simulink model "elec_a2d_sd_anti_alias_graph"  (R2020b)
settings: Solver=VariableStepAuto  StartTime=0.0  StopTime=60  MaxStep=3e-5  RelTol=1e-3  EnableMultiTasking=on
PreLoadFcn:
  | %% Global model parameters
  | fs = 1000; % A-to-D sampling rate
  | 
  | %% Filter design
  | f1 = 500; % Filter cut-off frequency
  | n = 4;    % Filter order
  | w1 = 2*pi*f1;
  | 
  | % [tmpB,tmpA] = besself(n,1); % Signal Processing Toolbox(TM)
  | tmpB = [0 0 0 0 1];
  | tmpA = [1.0000    3.1239    4.3916    3.2011    1.0000];
  | tmp_roots = roots(tmpA);
  | tcc1 = poly(tmp_roots(3:4));
  | a1 = tcc1(2);
  | b1 = tcc1(3);
  | tcc2 = poly(tmp_roots(1:2));
  | a2 = tcc2(2);
  | b2 = tcc2(3);
  | 
  | %% Filter implementation
  | R = 1e4;  % Resistance value
  | % Stage 1
  | C1 = a1/(2*b1);
  | C2 = 1/(b1*C1);
  | C1_1 = C1/( R*w1 );
  | C2_1 = C2/( R*w1 );
  | % Stage 2
  | C1 = a2/(2*b2);
  | C2 = 1/(b2*C1);
  | C1_2 = C1/( R*w1 );
  | C2_2 = C2/( R*w1 );
libraries: fl_lib x15, nesl_utility x4, ee_lib x1
CloseFcn:
  | try,close(h1_elec_a2d_sd_anti_alias),end
  | clear h1_elec_a2d_sd_anti_alias
  | 
  | 
  | clear simlog_elec_a2d_sd_anti_alias
  | clear logsout_elec_a2d_sd_anti_alias
  | clear C1 C1_1 C1_2 C2 C2_1 C2_2 R a1 a2 b1 b2 f1 fs n tcc1 tcc2 tmpA tmpB tmp_roots vOut w1
Description:
  | Analog Anti-Aliasing Filter
  | 
  | Copyright 2008-2018 The MathWorks, Inc.
settings Model: Creator=MathWorks  LastModifiedBy=dhrumilnaik
settings DataIOCC: MaxDataPoints=75000  SaveFormat=Array  SignalLoggingSaveFormat=ModelDataLogs  SaveOutput=off  SignalLogging=off  DSMLogging=off  SaveTime=off  ReturnWorkspaceOutputs=off  SignalLoggingName=logsout_elec_a2d_sd_anti_alias
settings OptimizationCC: ExpressionDepthLimit=2147483647  LifeSpan=inf
settings DebuggingCC: UnderspecifiedInitializationDetection=Classic  MergeDetectMultiDrivingBlocksExec=none  SolverPrmCheckMsg=warning  FcnCallInpInsideContextMsg=warning  StateNameClashWarn=warning  SFUnexpectedBacktrackingDiag=warning  SFNoUnconditionalDefaultTransitionDiag=warning  SFExecutionAtInitializationDiag=none  ArithmeticOperatorsInVariantConditions=warning
settings HardwareCC: ProdBitPerPointer=32  ProdBitPerSizeT=32  ProdBitPerPtrDiffT=32  ProdLargestAtomicFloat=None  ProdIntDivRoundTo=Undefined  ProdEndianess=Unspecified  ProdWordSize=32  ProdHWDeviceType=32-bit Generic
settings ModelReferenceCC: PropagateSignalLabelsOutOfModel=off
settings SFSimCC: SimUseLocalCustomCode=off  CustomCodeUndefinedFunction=UseInterfaceOnly
settings RTWCC: RTWUseLocalCustomCode=off
settings CodeAppCC: StateflowObjectComments=on
settings GRTTargetCC: TargetLangStandard=C89/C90 (ANSI)  CombineOutputUpdateFcns=off  GRTInterface=on
settings ConfigComp: CovMetricSettings=dw  CovSaveCumulativeToWorkspaceVar=on  CovSaveSingleToWorkspaceVar=on  CovExternalEMLEnable=off  CovSFcnEnable=off
settings SimscapeCC: SimscapeLogType=all  SimscapeLogSimulationStatistics=on  SimscapeLogName=simlog_elec_a2d_sd_anti_alias  SimscapeLogDataHistory=75000

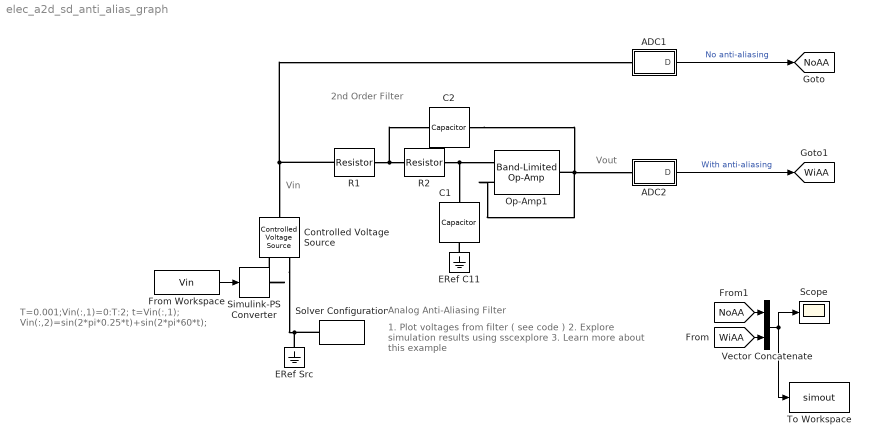
== system elec_a2d_sd_anti_alias_graph ==
  note: T=0.001;Vin(:,1)=0:T:2;
      |  t=Vin(:,1);
      | Vin(:,2)=sin(2*pi*0.25*t)+sin(2*pi*60*t);
  note: Vin
  note: 2nd Order Filter
  note: Analog Anti-Aliasing Filter
  note: 1. Plot voltages from filter ( see code )
      | 2. Explore simulation results using sscexplore
      | 3. Learn more about this example
  note: Vout
  " Scope" : Scope
  ADC1 : Subsystem  mask(ADC){fs=80, N=12, vmax=3.3, ileak=1e-9, C=10e-12}
      mask prompts: fs "Sampling rate (Hz)"; N "Number of bits"; vmax "Input voltage for max output (V)"; ileak "Leakage current (A)"; C "Pin capacitance (F)"
      mask help: Simplified analog-to-digital converter
  ADC2 : Subsystem  mask(ADC){fs=80, N=12, vmax=3.3, ileak=1e-9, C=10e-12}
      mask prompts: fs "Sampling rate (Hz)"; N "Number of bits"; vmax "Input voltage for max output (V)"; ileak "Leakage current (A)"; C "Pin capacitance (F)"
      mask help: Simplified analog-to-digital converter
  C1 : fl_lib/Electrical/Electrical Elements/Capacitor  c=0.1 uF  r=0 Ohm  g=0 1/Ohm  i_specify=off  i_priority=High  i=0 A  i_nominal_specify=off  i_nominal_unit=A  i_nominal_value=1  v_specify=off  v_priority=High  v=0 V  v_nominal_specify=off  v_nominal_unit=V  v_nominal_value=1  vc_specify=off  vc_priority=High  vc=0 V  vc_nominal_specify=off  vc_nominal_unit=V  vc_nominal_value=1
      settings: SourceProductName=Foundation Library
  C2 : fl_lib/Electrical/Electrical Elements/Capacitor  c=0.2 uF  r=0 Ohm  g=0 1/Ohm  i_specify=off  i_priority=High  i=0 A  i_nominal_specify=off  i_nominal_unit=A  i_nominal_value=1  v_specify=off  v_priority=High  v=0 V  v_nominal_specify=off  v_nominal_unit=V  v_nominal_value=1  vc_specify=off  vc_priority=High  vc=0 V  vc_nominal_specify=off  vc_nominal_unit=V  vc_nominal_value=1
      settings: SourceProductName=Foundation Library
  Controlled Voltage Source : fl_lib/Electrical/Electrical Sources/Controlled Voltage Source
  ERef C11 : fl_lib/Electrical/Electrical Elements/Electrical Reference
      settings: SourceProductName=Foundation Library
  ERef Src : fl_lib/Electrical/Electrical Elements/Electrical Reference
      settings: SourceProductName=Foundation Library
  From Workspace : FromWorkspace  VariableName=Vin
  Op-Amp1 : ee_lib/Integrated Circuits/Band-Limited Op-Amp  A=50000  Rin=6e+6 Ohm  Rout=100 Ohm  Vmin=-15 V  Vmax=15 V  Vdotmax=0.7e6 V/s  f=1.5e+6 Hz  V0=0 V
      settings: SourceProductBaseCode=PS
  R1 : fl_lib/Electrical/Electrical Elements/Resistor  R=62 kOhm  i_specify=off  i_priority=High  i=0 A  i_nominal_specify=off  i_nominal_unit=A  i_nominal_value=1  v_specify=off  v_priority=High  v=0 V  v_nominal_specify=off  v_nominal_unit=V  v_nominal_value=1
      settings: SourceProductName=Foundation Library
  R2 : fl_lib/Electrical/Electrical Elements/Resistor  R=62 kOhm  i_specify=off  i_priority=High  i=0 A  i_nominal_specify=off  i_nominal_unit=A  i_nominal_value=1  v_specify=off  v_priority=High  v=0 V  v_nominal_specify=off  v_nominal_unit=V  v_nominal_value=1
      settings: SourceProductName=Foundation Library
  Simulink-PS Converter : nesl_utility/Simulink-PS Converter  PhysicalDomain=network_engine_domain  SubClassName=ps_input  LeftPortType=input  RightPortType=output  PseudoPeriodic=off  Frequencies=[]  NoiseDistribution=none  NoiseParameters=[]  Unit=1  AffineConversion=off  FilteringAndDerivatives=zero  SimscapeFilterOrder=1  InputFilterTimeConstant=.001  UdotUserProvided=0
  Solver Configuration : nesl_utility/Solver Configuration  PhysicalDomain=network_engine_domain  SubClassName=solver  LeftPortType=input  RightPortType=generic  Tones=[]  Harmonics=[]  SimulateNoise=off  Profile=off  UseLocalSampling=off  EnableSwitchedLinearOptims=on  FrequencyDomain=off  UseCCode=off  RelTol=0.001  AbsTol=1e-06  MinStep=1e-09  ToWorkspace=off  RevertToSquareIcSolve=off  NumHomotopyIterations=100  PhasorMode=off  PhasorModeNumHarmonics=1  DoDC=off  ResidualTolerance=1e-9  UseLocalSolver=off  LocalSolverChoice=NE_BACKWARD_EULER_ADVANCER  LocalSolverSampleTime=1e-6  DoFixedCost=off  MaxNonlinIter=3  MaxModeIter=2  ComputeImpulses=off  ImpulseIterations=2  LinearAlgebra=auto  EquationFormulation=NE_TIME_EF  DelaysMemoryBudget=1024  AutomaticFiltering=on  FilteringTimeConstant=0.001  PartitionStorageMethod=AS_NEEDED  PartitionMemoryBudget=1024  PartitionMethod=FAST
  To Workspace : ToWorkspace  VariableName=simout  SaveFormat=Timeseries  SampleTime=-1
  Vector Concatenate : Concatenate  Mode=Multidimensional array  ConcatenateDimension=2
  tag scope: NoAA=global, WiAA=global
  wires:
  Vector Concatenate/1 -> To Workspace/1, " Scope"/1
  ADC1/1(D) -> [NoAA]  "No anti-aliasing"
  ADC2/1(D) -> [WiAA]  "With anti-aliasing"
  [WiAA] -> Vector Concatenate/2
  [NoAA] -> Vector Concatenate/1
  From Workspace/1 -> Simulink-PS Converter/1
  connections:
  ERef Src/LConn1 -- Controlled Voltage Source/RConn2 -- Solver Configuration/RConn1
  R2/RConn1 -- C1/LConn1 -- Op-Amp1/LConn1
  R1/RConn1 -- C2/LConn1 -- R2/LConn1
  Op-Amp1/RConn1 -- ADC2/LConn1 -- C2/RConn1 -- Op-Amp1/LConn2
  ERef C11/LConn1 -- C1/RConn1
  R1/LConn1 -- Controlled Voltage Source/LConn1 -- ADC1/LConn1
  Simulink-PS Converter/RConn1 -- Controlled Voltage Source/RConn1

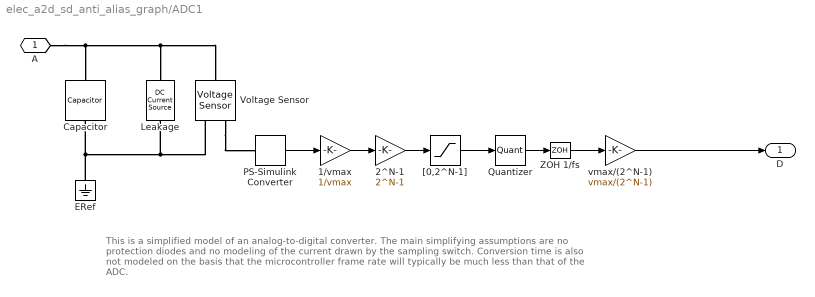
== system elec_a2d_sd_anti_alias_graph/ADC1 ==
  note: This is a simplified model of an analog-to-digital converter. The main simplifying assumptions
      | are no protection diodes and no modeling of the current drawn by the sampling switch.
      | Conversion time is also not modeled on the basis that the microcontroller frame rate will
      | typically be much less than that of the ADC.
  1/vmax : Gain  Gain=1/vmax
  2^N-1 : Gain  Gain=2^N-1
  Capacitor : fl_lib/Electrical/Electrical Elements/Capacitor  c=1e-6 F  r=1e-6 Ohm  g=0 1/Ohm  i_specify=off  i_priority=High  i=0 A  i_nominal_specify=off  i_nominal_unit=A  i_nominal_value=1  v_specify=off  v_priority=High  v=0 V  v_nominal_specify=off  v_nominal_unit=V  v_nominal_value=1  vc_specify=on  vc_priority=High  vc=0 V  vc_nominal_specify=off  vc_nominal_unit=V  vc_nominal_value=1
      settings: SourceProductName=Foundation Library
  ERef : fl_lib/Electrical/Electrical Elements/Electrical Reference
      settings: SourceProductName=Foundation Library
  Leakage : fl_lib/Electrical/Electrical Sources/DC Current Source  i0=ileak A
      settings: SourceProductName=Foundation Library  InternalSimscapePortConfiguration="{\"Bottom\":[],\"Left\":[{\"id\":\"p\",\"label\":\"\",\"type\":\"foundation.electrical.electrical\"}],\"Right\":[{\"id\":\"n\",\"label\":\"\",\"type\":\"foundation.electrical.electrical\"}],\"Top\":[]}"
  PS-Simulink Converter : nesl_utility/PS-Simulink Converter  PhysicalDomain=network_engine_domain  SubClassName=ps_output  LeftPortType=input  RightPortType=output  PseudoPeriodic=off  Frequencies=[]  Unit=V  AffineConversion=off
  Quantizer : Quantizer
  Voltage Sensor : fl_lib/Electrical/Electrical Sensors/Voltage Sensor
      settings: SourceProductName=Foundation Library
  ZOH 1/fs : ZeroOrderHold  SampleTime=1/fs
  "[0,2^N-1]" : Saturate  UpperLimit=2^N-1  LowerLimit=0
  vmax/(2^N-1) : Gain  Gain=vmax/(2^N-1)
  A : PMIOPort  Side=Left
  D : Outport  VectorParamsAs1DForOutWhenUnconnected=off
  wires:
  "[0,2^N-1]"/1 -> Quantizer/1
  1/vmax/1 -> 2^N-1/1
  2^N-1/1 -> "[0,2^N-1]"/1
  PS-Simulink Converter/1 -> 1/vmax/1
  ZOH 1/fs/1 -> vmax/(2^N-1)/1
  Quantizer/1 -> ZOH 1/fs/1
  vmax/(2^N-1)/1 -> D/1
  connections:
  A/RConn1 -- Voltage Sensor/LConn1 -- Leakage/RConn1 -- Capacitor/LConn1
  ERef/LConn1 -- Voltage Sensor/RConn2 -- Leakage/LConn1 -- Capacitor/RConn1
  Voltage Sensor/RConn1 -- PS-Simulink Converter/LConn1

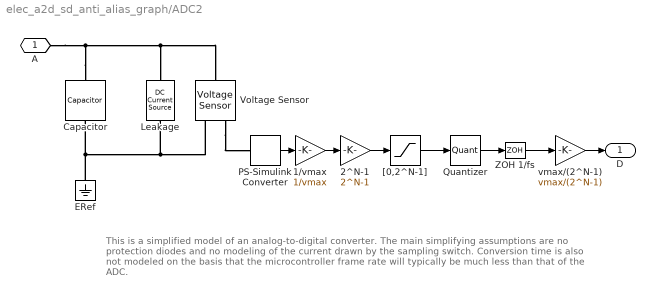
== system elec_a2d_sd_anti_alias_graph/ADC2 ==
  note: This is a simplified model of an analog-to-digital converter. The main simplifying assumptions
      | are no protection diodes and no modeling of the current drawn by the sampling switch.
      | Conversion time is also not modeled on the basis that the microcontroller frame rate will
      | typically be much less than that of the ADC.
  1/vmax : Gain  Gain=1/vmax
  2^N-1 : Gain  Gain=2^N-1
  Capacitor : fl_lib/Electrical/Electrical Elements/Capacitor  c=1e-6 F  r=1e-6 Ohm  g=0 1/Ohm  i_specify=off  i_priority=High  i=0 A  i_nominal_specify=off  i_nominal_unit=A  i_nominal_value=1  v_specify=off  v_priority=High  v=0 V  v_nominal_specify=off  v_nominal_unit=V  v_nominal_value=1  vc_specify=on  vc_priority=High  vc=0 V  vc_nominal_specify=off  vc_nominal_unit=V  vc_nominal_value=1
      settings: SourceProductName=Foundation Library
  ERef : fl_lib/Electrical/Electrical Elements/Electrical Reference
      settings: SourceProductName=Foundation Library
  Leakage : fl_lib/Electrical/Electrical Sources/DC Current Source  i0=ileak A
      settings: SourceProductName=Foundation Library  InternalSimscapePortConfiguration="{\"Bottom\":[],\"Left\":[{\"id\":\"p\",\"label\":\"\",\"type\":\"foundation.electrical.electrical\"}],\"Right\":[{\"id\":\"n\",\"label\":\"\",\"type\":\"foundation.electrical.electrical\"}],\"Top\":[]}"
  PS-Simulink Converter : nesl_utility/PS-Simulink Converter  PhysicalDomain=network_engine_domain  SubClassName=ps_output  LeftPortType=input  RightPortType=output  PseudoPeriodic=off  Frequencies=[]  Unit=V  AffineConversion=off
  Quantizer : Quantizer
  Voltage Sensor : fl_lib/Electrical/Electrical Sensors/Voltage Sensor
      settings: SourceProductName=Foundation Library
  ZOH 1/fs : ZeroOrderHold  SampleTime=1/fs
  "[0,2^N-1]" : Saturate  UpperLimit=2^N-1  LowerLimit=0
  vmax/(2^N-1) : Gain  Gain=vmax/(2^N-1)
  A : PMIOPort  Side=Left
  D : Outport  VectorParamsAs1DForOutWhenUnconnected=off
  wires:
  vmax/(2^N-1)/1 -> D/1
  Quantizer/1 -> ZOH 1/fs/1
  ZOH 1/fs/1 -> vmax/(2^N-1)/1
  PS-Simulink Converter/1 -> 1/vmax/1
  2^N-1/1 -> "[0,2^N-1]"/1
  1/vmax/1 -> 2^N-1/1
  "[0,2^N-1]"/1 -> Quantizer/1
  connections:
  Voltage Sensor/RConn1 -- PS-Simulink Converter/LConn1
  Leakage/LConn1 -- ERef/LConn1 -- Capacitor/RConn1 -- Voltage Sensor/RConn2
  Capacitor/LConn1 -- Leakage/RConn1 -- Voltage Sensor/LConn1 -- A/RConn1
